simulink model "Real_Data__Collection"  (R2023a)
settings: Solver=FixedStepAuto  StartTime=0.0  StopTime=20  FixedStep=0.05  RelTol=1e-3  EnableMultiTasking=on
libraries: arduinolib x3, arduinosensorlib x1
settings Model: ExtModeTrigDuration=2  Creator=RAOUF  LastModifiedBy=RAOUF
settings DataIOCC: SaveFormat=StructureWithTime  ReturnWorkspaceOutputs=off
settings OptimizationCC: EnhancedBackFolding=on  PassReuseOutputArgsAs=Individual arguments  ZeroExternalMemoryAtStartup=off  ZeroInternalMemoryAtStartup=off  MaxStackSize=64  OptimizeBlockOrder=speed  DifferentSizesBufferReuse=on  OptimizationCustomize=off  EfficientTunableParamExpr=on
settings DebuggingCC: ParameterTunabilityLossMsg=error
settings HardwareCC: ProdBitPerInt=16  ProdBitPerPointer=16  ProdBitPerSizeT=16  ProdBitPerPtrDiffT=16  ProdLargestAtomicFloat=None  ProdWordSize=8  ProdHWDeviceType=Atmel->AVR
settings SFSimCC: MATLABDynamicMemAlloc=off
settings RTWCC: Description=Embedded Coder  SystemTargetFile=ert.tlc  HardwareBoard=Arduino Uno  TemplateMakefile=ert_default_tmf  Toolchain=Arduino AVR  BuildConfiguration=Faster Runs
settings CodeAppCC: ForceParamTrailComments=on  IgnoreCustomStorageClasses=off  OperatorAnnotations=on  SimulinkDataObjDesc=on  SFDataObjDesc=on  InsertBlockDesc=on
settings ERTTargetCC: SupportContinuousTime=on  SupportVariableSizeSignals=on  ExtModeTransport=3  ExtModeStaticAlloc=on  ExtModeAutomaticAllocSize=off  ExtModeStaticAllocSize=250  ExtModeMexFile=ext_xcp  ExtModeIntrfLevel=Level2 - Open

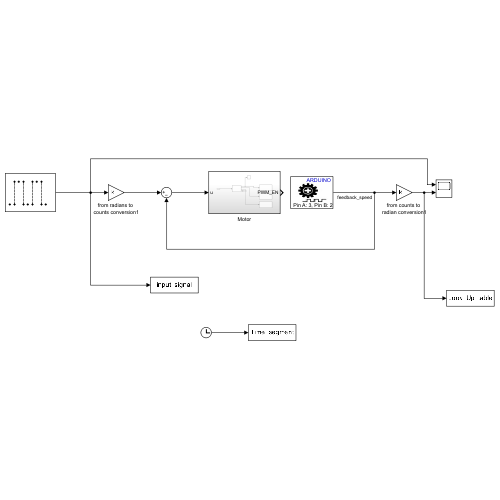
[thumbnail: Simulink's stored preview of the top-level diagram]
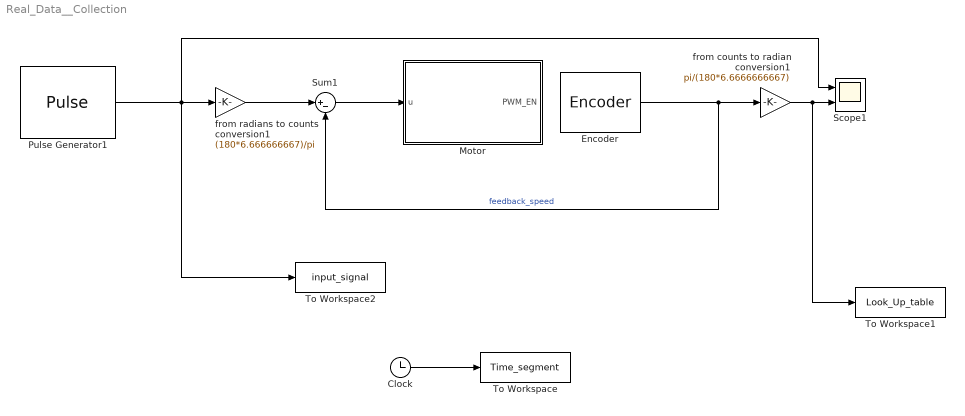
== system Real_Data__Collection ==
  Clock : Clock
  Encoder : arduinosensorlib/Encoder  InputA=3  InputB=2  Mode=No reset  SampleTime=-1
  Motor : Subsystem
  Pulse Generator1 : DiscretePulseGenerator  Amplitude=60  Period=40  PulseWidth=20  PhaseDelay=5  SampleTime=0.05
  Scope1 : Scope  NumInputPorts=2
  Sum1 : Sum  Inputs=|+-
  To Workspace : ToWorkspace  VariableName=Time_segment  SampleTime=-1
      settings: Save2DSignal=2-D array (concatenate along first dimension)
  To Workspace1 : ToWorkspace  VariableName=Look_Up_table  SampleTime=-1
      settings: Save2DSignal=2-D array (concatenate along first dimension)
  To Workspace2 : ToWorkspace  VariableName=input_signal  SampleTime=-1
      settings: Save2DSignal=2-D array (concatenate along first dimension)
  from counts to radian conversion1 : Gain  Gain=pi/(180*6.6666666667)
  from radians to counts conversion1 : Gain  Gain=(180*6.666666667)/pi
  wires:
  Clock/1 -> To Workspace/1
  Pulse Generator1/1 -> from radians to counts conversion1/1, Scope1/1, To Workspace2/1
  Encoder/1 -> from counts to radian conversion1/1, Sum1/2  "feedback_speed"
  Sum1/1 -> Motor/1(u)
  from radians to counts conversion1/1 -> Sum1/1
  from counts to radian conversion1/1 -> To Workspace1/1, Scope1/2

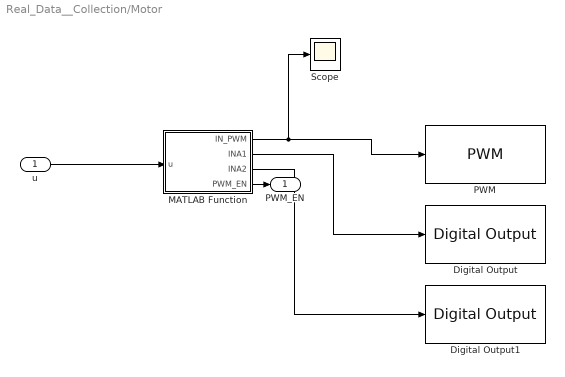
== system Real_Data__Collection/Motor ==
  u : Inport
  Digital Output : arduinolib/Digital Output  pinNumber=9  Direction=output  blockPlatform=arduino
  Digital Output1 : arduinolib/Digital Output  pinNumber=10  Direction=output  blockPlatform=arduino
  MATLAB Function : MATLAB Function  TreatAsAtomicUnit=on
  PWM : arduinolib/PWM  pinNumber=5  frequencyType=Default  desiredFrequency=490.2  achievableFrequency=490.2
  Scope : Scope
  PWM_EN : Outport
  wires:
  MATLAB Function/2(INA1) -> Digital Output/1
  MATLAB Function/1(IN_PWM) -> Scope/1, PWM/1
  MATLAB Function/3(INA2) -> Digital Output1/1
  MATLAB Function/4(PWM_EN) -> PWM_EN/1
  u/1 -> MATLAB Function/1(u)

== matlab function Real_Data__Collection/Motor/MATLAB Function ==
  data: u input; IN_PWM output; INA1 output; INA2 output; PWM_EN output
function [IN_PWM,INA1,INA2,PWM_EN] = fcn(u)

PWM_EN = u;
IN_PWM=abs(u);
if u<0
    INA1=0;
    INA2=1;
elseif u>0
    INA1=1;
    INA2=0;
else
    INA1=0;
    INA2=0;
end
